simulink model "test"  (R2021b)
settings: Solver=FixedStepAuto  StartTime=0.0  StopTime=inf  FixedStep=0.01  RelTol=1e-3
undefined symbols (not defined in the file or in its folder): X, Y
libraries: robotlib x3
settings Model: Creator=cheng  LastModifiedBy=cheng

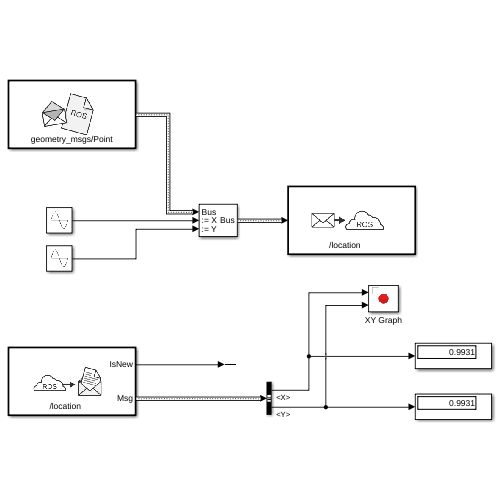
[thumbnail: Simulink's stored preview of the top-level diagram]
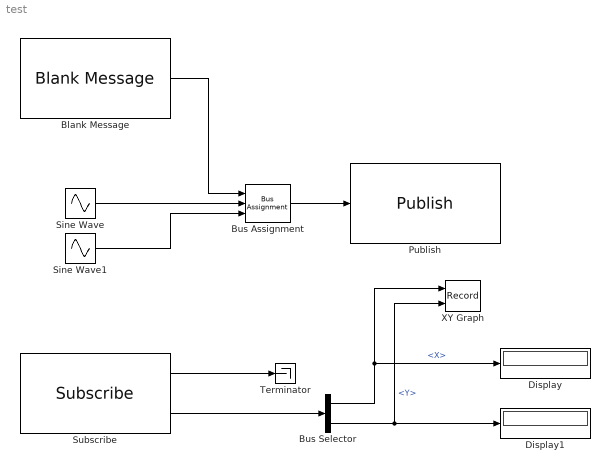
== system test ==
  Blank Message : robotlib/Blank Message  messageClass=Message  entityType=geometry_msgs/Point  messageType=geometry_msgs/Point  SampleTime=inf  legacyBusStruct=off
  Bus Assignment : BusAssignment  AssignedSignals=X,Y
  Bus Selector : BusSelector  OutputSignals=X,Y
  Display : Display
  Display1 : Display
  Publish : robotlib/Publish  topicSource=Specify your own  topic=/location  messageType=geometry_msgs/Point  legacyBusStruct=off  messageQueueLength=1
  Sine Wave : Sin  Phase=-pi/2  SampleTime=0
  Sine Wave1 : Sin  Phase=-pi/2  SampleTime=0
  Subscribe : robotlib/Subscribe  topicSource=Specify your own  topic=/location  messageType=geometry_msgs/Point  SampleTime=-1  legacyBusStruct=off  messageQueueLength=1
  Terminator : Terminator
  XY Graph : Record  FileSettingsInternal="{\"entries\":[{\"content\":{\"excelSettings\":{\"content\":{},\"type\":\"Streamout.ExcelSettings\"}},\"type\":\"Streamout.FileSettingStorage\",\"uuid\":\"3838be85-1f1c-4b99-b4a7-3625c71cf0da\"}],\"packageUris\":[\"http://schema.mathworks.com/mf0/streamout_blocks/R2020a\"],\"version\":\"1.0\"}"  Layout=[1 1]  SignalsInternal="{\"entries\":[{\"content\":{\"signals\":[{\"content\":{\"blockPath\":[\"test/XY Graph\"],\"channel\":[],\"dimensions\":[1],\"domain\":\"test/XY Graph\",\"lineColor\":\"#fe330a\",\"plots\":[],\"port\":1,\"sid\":[\"\"],\"signalID\":1287,\"signalName\":\"<X>\"},\"type\":\"RecordBlkView.Signal\",\"uuid\":\"6a83e0ba-4536-4e51-8a87-4660c02c7405\"},{\"content\":{\"blockPath\":[\"test/XY Graph\"],\"channel\":[],\"dimensions\":[1],\"domain\":\"test/XY Graph\",\"lineColor\":\"#22b573\",\"plots\":[],\"port\":2,\"sid\":[\"\"],\"signalID\":1291,\"signalName\":\"<Y>\"},\"type\":\"RecordBlkView.Signal\",\"uuid\":\"1b3b6f35-997d-4057-a577-e7c8d15fa29c\"}]},\"type\":\"RecordBlkView.InputSignals\",\"uuid\":\"129e22e1-0d89-4664-8236-bc3a07bba35b\"}],\"packageUris\":[\"http://schema.mathworks.com/mf0/streamout_blocks/R2020a\"],\"version\":\"1.0\"}"  VisualizationBindings="{\"xyplotplugin\":{\"info\":[{\"series\":[],\"subplotID\":1}]}}"  CompatibilityTag=XY
  wires:
  Blank Message/1 -> Bus Assignment/1
  Bus Assignment/1 -> Publish/1
  Sine Wave/1 -> Bus Assignment/2
  Sine Wave1/1 -> Bus Assignment/3
  Subscribe/2 -> Bus Selector/1
  Subscribe/1 -> Terminator/1
  Bus Selector/1 -> Display/1, XY Graph/1  "<X>"
  Bus Selector/2 -> XY Graph/2, Display1/1  "<Y>"
